simulink model "p1"  (R2016a)
settings: Solver=VariableStepAuto  StartTime=0.0  StopTime=10  RelTol=1e-3
undefined symbols (not defined in the file or in its folder): fdesignblkfcn, gcbh
libraries: simrfV2elements x2, simrfV2util1 x2, simrfV2sources1 x2, fl_lib x1
settings Model: Creator=eia14hx  LastModifiedBy=eia14hx

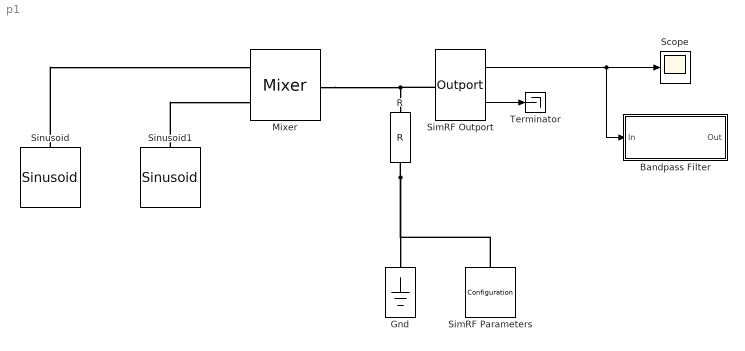
== system p1 ==
  Bandpass Filter : Subsystem  DialogController=fdesignblkfcn  InitFcn=fdesignblkfcn(gcbh, {'InitFcn'});  mask(Bandpass Filter){}
      mask help: Design a bandpass filter
      settings: CopyFcn=fdesignblkfcn(gcbh, {'CopyFcn'});
      mask Help: helpview(mapfilelocation('dsp'), 'dspbandpassfilter');
      mask Display: disp('Bandpass');
  Gnd : fl_lib/Electrical/Electrical Elements/Electrical Reference
  Mixer : simrfV2elements/Mixer  classname=mixer  Source_linear_gain=Available power gain  linear_gain=0 dB  Zin=50  Zout=50  ZLO=inf  Source_Poly=Even and odd order  Poly_Coeffs=0  IPType=Output  IP2=Inf dBm  IP3=Inf dBm  P1dB=Inf dBm  Psat=Inf dBm  Gcomp=Inf dBm  NF=0  InternalGrounding=on
  R : simrfV2elements/R  classname=resistor  Resistance=50 Ohm  AddNoise=on
  Scope : Scope
  SimRF Outport : simrfV2util1/Outport  SensorType=Ideal voltage  OutputFormat=In-phase and Quadrature Baseband  CarrierFreq=108e3-9.960 kHz  ZL=Inf  InternalGrounding=on  StepSize=-1 s  AutoStep=off
  SimRF Parameters : simrfV2util1/Configuration  AutoFreq=on  Tones="[0.00996           108] MHz"  Harmonics="[5  5]"  NormalizeCarrierPower=on  SolverType=Auto  StepSize=1e-3 s  AddNoise=off  Temperature=293.15 K  SolverDelFlag=0
  Sinusoid : simrfV2sources1/Sinusoid  SineSourceType=Ideal voltage  VO_I=0 V  IO_I=0 A  VO_Q=0 V  IO_Q=0 A  VA_I=1 V  IA_I=0 A  VA_Q=0 V  IA_Q=0 A  Fmod=30 Hz  TD=0 s  CarrierFreq=9960 Hz  InternalGrounding=on
  Sinusoid1 : simrfV2sources1/Sinusoid  SineSourceType=Ideal voltage  VO_I=0 V  IO_I=0 A  VO_Q=0 V  IO_Q=0 A  VA_I=1 V  IA_I=0 A  VA_Q=0 V  IA_Q=0 A  Fmod=30 Hz  TD=1/30 s  CarrierFreq=108e6 Hz  InternalGrounding=on
  Terminator : Terminator
  wires:
  SimRF Outport/1 -> Bandpass Filter/1(In), Scope/1
  SimRF Outport/2 -> Terminator/1
  connections:
  Sinusoid1/LConn1 -- Mixer/LConn2
  Sinusoid/LConn1 -- Mixer/LConn1
  R/RConn1 -- Gnd/LConn1 -- SimRF Parameters/LConn1
  Mixer/RConn1 -- SimRF Outport/LConn1 -- R/LConn1

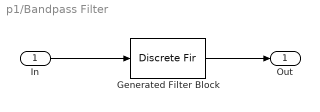
== system p1/Bandpass Filter ==
  In : Inport
  Generated Filter Block : DiscreteFir  Tag=BlockMethodSubSystem  Coefficients=[-0.0008992291487744296 0.0016414518747943749 0.0031352071842225397 -0.0040707550828814922 -0.0063731852227904111 0.0074874286806090491 0.0098354319566295711 -0.010189316513446216 -0.011302794465874122 0.0096929185841818435 0.0079428653987464216 -0.0031368247881221642 0.0028299878877943137 -0.011508674243001471 -0.022080136219461581 0.034245325424507672 0.048356661648905473 -0.062355369169884239 -0.077503478162593897 0.090687768153125653 0.10353171105844157 -0.11297860084229834 -0.12035866024978455 0.12379360801539134 0.12379360801539134 -0.12035866024978455 -0.11297860084229834 0.10353171105844157 0.090687768153125653 -0.077503478162593897 -0.062355369169884239 0.048356661648905473 0.034245325424507672 -0.022080136219461581 -0.011508674243001471 0.0028299878877943137 -0.0031368247881221642 0.0079428653987464216 0.0096929185841818435 -0.011302794465874122 -0.010189316513446216 0.0098354319566295711 0.0074874286806090491 -0.0063731852227904111 -0.0040707550828814922 0.0031352071842225397 0.0016414518747943749 -0.0008992291487744296]  InputProcessing=Columns as channels (frame based)
  Out : Outport
  wires:
  In/1 -> Generated Filter Block/1
  Generated Filter Block/1 -> Out/1
